simulink model "laba5_QPSK"  (Simulink 7.5)
settings: Solver=ode45  StartTime=0.0  StopTime=10.0  RelTol=1e-3
libraries: dspbuff3 x3, commsequence2 x1, commseqgen2 x1, commutil2 x1
settings Model: Creator=Lenovo  LastModifiedBy=Lenovo

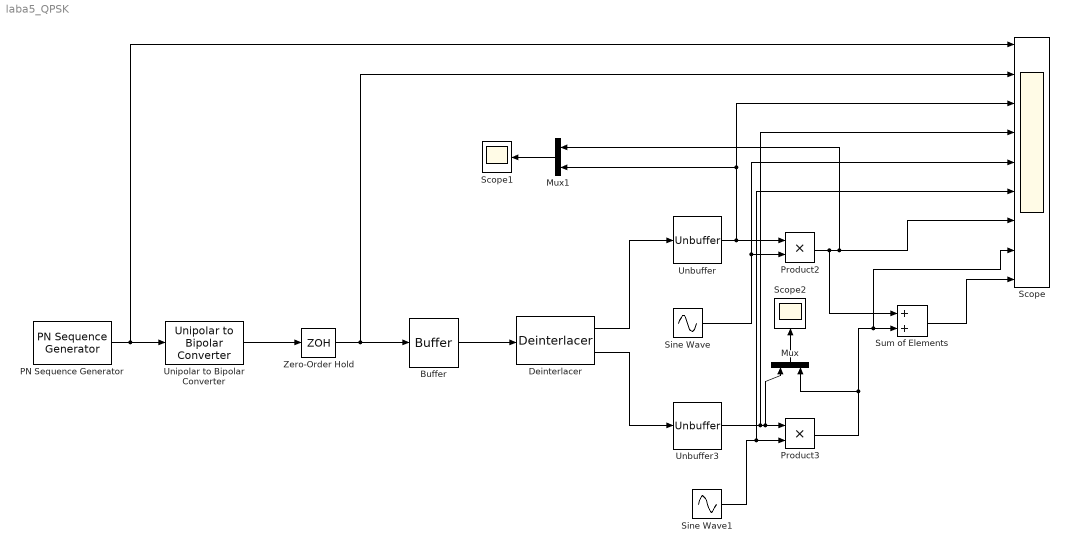
== system laba5_QPSK ==
  Buffer : dspbuff3/Buffer  N=2  V=0  ic=0
  Deinterlacer : commsequence2/Deinterlacer
  Mux : Mux  Inputs=2
  Mux1 : Mux  Inputs=2
  PN Sequence Generator : commseqgen2/PN Sequence Generator  poly=[1 0 0 0 0 1 1]  ini_sta=[0 0 0 0 0 1]  outBitMaskSource=Input port  shift=0  Ts=1/1200  frameBased=off  sampPerFrame=1  reset=off  bitPackedOutputs=off  outDataType=double  numPackedBits=8  bitPackDataSigned=off  bitPackedOutDType=double
  Product2 : Product  OutDataType=fixdt(1, 16)  OutScaling=2^0  RndMeth=Zero
  Product3 : Product  OutDataType=fixdt(1, 16)  OutScaling=2^0  RndMeth=Zero
  Scope : Scope  NumInputPorts=9
      settings: TickLabels=on  TimeRange=12  YMin=-5~-5~-5~-5~-5~-5~-5~-5~-5  YMax=5~5~5~5~5~5~5~5~5  SaveName=ScopeData2
  Scope1 : Scope
  Scope2 : Scope
  Sine Wave : Sin  Amplitude=1  Bias=0  Frequency=753600  Phase=?pi/2  Samples=10  SampleTime=0  Offset=0
  Sine Wave1 : Sin  Amplitude=1  Bias=0  Frequency=753600  Phase=0  Samples=10  SampleTime=0  Offset=0
  Sum of Elements : Sum  OutDataType=fixdt(1, 16)  OutScaling=2^-10
  Unbuffer : dspbuff3/Unbuffer  ic=0
  Unbuffer3 : dspbuff3/Unbuffer  ic=0
  Unipolar to Bipolar Converter : commutil2/Unipolar to Bipolar Converter  SystemSampleTime=-1  M=2  polarity=Positive  dataType=Inherit via internal rule
  Zero-Order Hold : ZeroOrderHold
  wires:
  PN Sequence Generator/1 -> Unipolar to Bipolar Converter/1, Scope/1
  Unipolar to Bipolar Converter/1 -> Zero-Order Hold/1
  Zero-Order Hold/1 -> Buffer/1, Scope/2
  Buffer/1 -> Deinterlacer/1
  Unbuffer/1 -> Product2/1, Scope/3, Mux1/2
  Unbuffer3/1 -> Scope/4, Product3/1, Mux/1
  Deinterlacer/1 -> Unbuffer/1
  Deinterlacer/2 -> Unbuffer3/1
  Mux/1 -> Scope2/1
  Product3/1 -> Mux/2, Sum of Elements/2, Scope/8
  Mux1/1 -> Scope1/1
  Sum of Elements/1 -> Scope/9
  Sine Wave/1 -> Scope/5, Product2/2
  Sine Wave1/1 -> Product3/2, Scope/6
  Product2/1 -> Scope/7, Mux1/1, Sum of Elements/1
